simulink model "VERIFICATION_EMACE_APP"  (R2021b)
settings: Solver=FixedStepDiscrete  StartTime=0.0  StopTime=10  FixedStep=sampleTime.model  RelTol=1e-3
undefined symbols (not defined in the file or in its folder): sampleTime
libraries: EMACE_APP x1, simulink x1
settings Model: Creator=ACH  LastModifiedBy=ACH

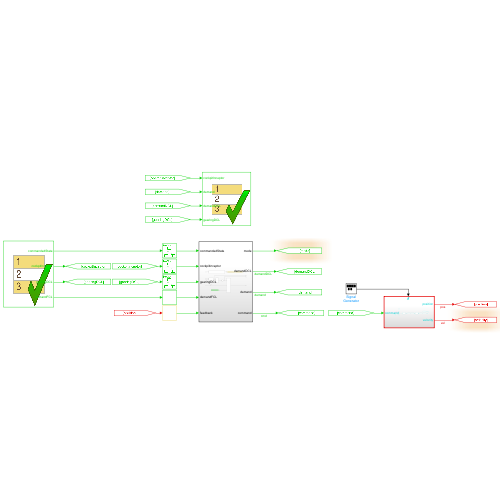
[thumbnail: Simulink's stored preview of the top-level diagram]
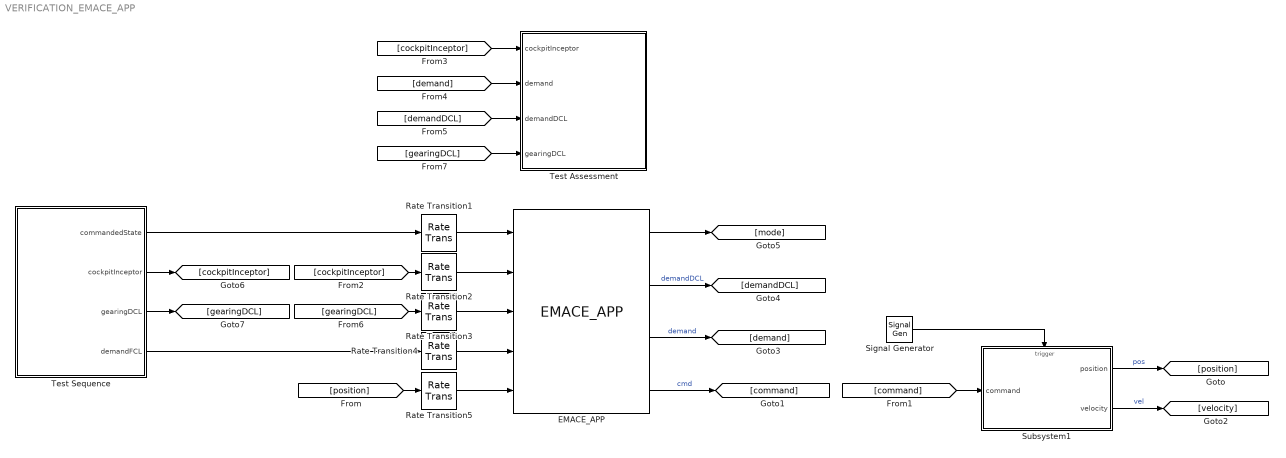
== system VERIFICATION_EMACE_APP ==
  EMACE_APP : EMACE_APP/EMACE_APP  SystemSampleTime=-1  VariantActivationTime=update diagram  Latency=0  AutoFrameSizeCalculation=off
  Rate Transition{1..5} (5 alike) : RateTransition  OutPortSampleTime=sampleTime.digital
  Signal Generator : SignalGenerator  WaveForm=square  Frequency=1/sampleTime.hardware  Units=rad/sec
  Subsystem1 : Subsystem
  Test Assessment : Test Sequence  TreatAsAtomicUnit=on
  Test Sequence : Test Sequence  TreatAsAtomicUnit=on
  wires:
  EMACE_APP/4 -> [command]  "cmd"
  [command] -> Subsystem1/1(command)
  Subsystem1/1(position) -> [position]  "pos"
  Test Sequence/1(commandedState) -> Rate Transition1/1
  Signal Generator/1 -> Subsystem1/Trigger
  Subsystem1/2(velocity) -> [velocity]  "vel"
  Test Sequence/3(gearingDCL) -> [gearingDCL]
  Test Sequence/4(demandFCL) -> Rate Transition4/1
  Rate Transition1/1 -> EMACE_APP/1
  Rate Transition2/1 -> EMACE_APP/2
  Rate Transition3/1 -> EMACE_APP/3
  Rate Transition4/1 -> EMACE_APP/4
  Rate Transition5/1 -> EMACE_APP/5
  [position] -> Rate Transition5/1
  EMACE_APP/3 -> [demand]  "demand"
  EMACE_APP/2 -> [demandDCL]  "demandDCL"
  EMACE_APP/1 -> [mode]
  Test Sequence/2(cockpitInceptor) -> [cockpitInceptor]
  [cockpitInceptor] -> Rate Transition2/1
  [cockpitInceptor] -> Test Assessment/1(cockpitInceptor)
  [demand] -> Test Assessment/2(demand)
  [demandDCL] -> Test Assessment/3(demandDCL)
  [gearingDCL] -> Rate Transition3/1
  [gearingDCL] -> Test Assessment/4(gearingDCL)

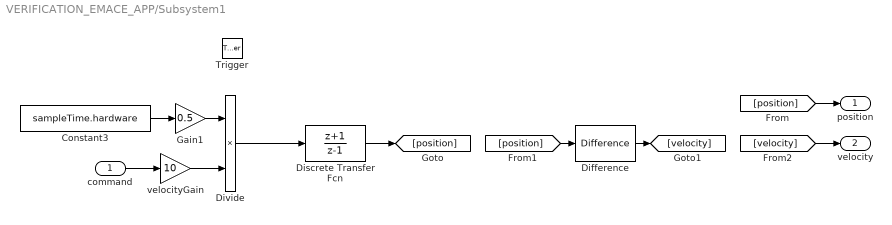
== system VERIFICATION_EMACE_APP/Subsystem1 ==
  command : Inport
  Trigger : TriggerPort  VariantControl=(inherit)  PortDimensions=1
  Constant3 : Constant  Value=sampleTime.hardware
  Difference : simulink/Discrete/Difference  ICPrevInput=0.0  OutMin=[]  OutMax=[]  OutDataType=fixdt(1, 16)  OutScaling=2^-10  DoSatur=off
  Discrete Transfer Fcn : DiscreteTransferFcn  Numerator=[1 1]  Denominator=[1 -1]
  Divide : Product  Inputs=**
  Gain1 : Gain  Gain=0.5
  velocityGain : Gain  Gain=10
  position : Outport
  velocity : Outport  Port=2
  wires:
  command/1 -> velocityGain/1
  Gain1/1 -> Divide/1
  Constant3/1 -> Gain1/1
  Divide/1 -> Discrete Transfer Fcn/1
  Discrete Transfer Fcn/1 -> [position]
  [position] -> position/1
  [position] -> Difference/1
  Difference/1 -> [velocity]
  [velocity] -> velocity/1
  velocityGain/1 -> Divide/2

== stateflow chart VERIFICATION_EMACE_APP/Test Assessment ==
  state step_1
    verify(abs(demand) < abs(cockpitInceptor*gearingDCL) + 0.01);
    verify(demandDCL < 0.01);
  (default) -> step_1
  data: cockpitInceptor input; demand input; demandDCL input; gearingDCL input

== stateflow chart VERIFICATION_EMACE_APP/Test Sequence ==
  state step_1
    commandedState = 1;
    cockpitInceptor = 10*sin(2*pi*t);
    gearingDCL = 0.354;
    demandFCL = 0;
  state step_2
    commandedState = 1;
    cockpitInceptor = 0;
    gearingDCL = 0.354;
    demandFCL = 0;
  (default) -> step_1
  step_1 -> step_2 : [
      | after(5,sec)
      | ]
  data: commandedState output; cockpitInceptor output; gearingDCL output; demandFCL output
